simulink model "sf_multfuncout"  (Simulink 7.6)
settings: Solver=ode45  StartTime=0.0  StopTime=30  MaxStep=1  RelTol=1e-3
settings Model: Creator=The MathWorks Inc.  CovMetricSettings=dcmtr  ExtModeAutoUpdateStatusClock=off
settings OptimizationCC: BooleanDataType=off  InlineInvariantSignals=on  InitFltsAndDblsToZero=on  EfficientMapNaN2IntZero=off
settings DebuggingCC: SaveWithParameterizedLinksMsg=none  SignalResolutionControl=TryResolveAllWithWarning  SolverPrmCheckMsg=none  MultiTaskDSMMsg=warning  MultiTaskCondExecSysMsg=none  StrictBusMsg=None
settings HardwareCC: TargetUnknown=on
settings SFSimCC: SimParseCustomCode=off
settings RTWCC: IncludeERTFirstTime=on
settings GRTTargetCC: TargetFcnLib=ansi_tfl_tmw.mat

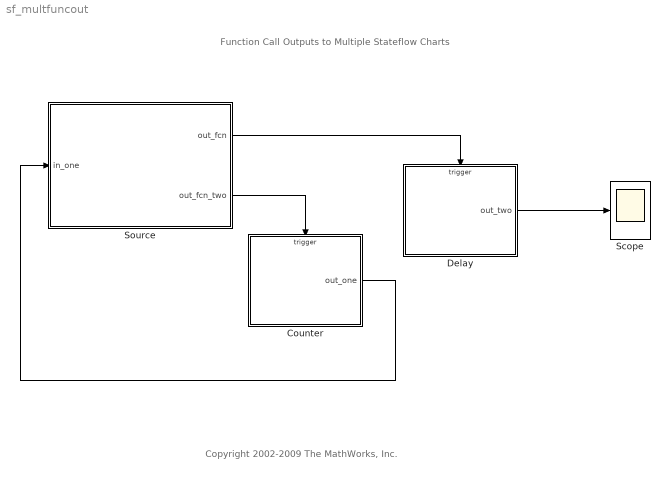
== system sf_multfuncout ==
  note: Function Call Outputs to Multiple Stateflow Charts
  note: Copyright 2002-2009 The MathWorks, Inc.
  Counter : Stateflow chart  TreatAsAtomicUnit=on
  Delay : Stateflow chart  TreatAsAtomicUnit=on
  Scope : Scope
      settings: TimeRange=30  YMin=0  YMax=7
  Source : Stateflow chart  TreatAsAtomicUnit=on
  wires:
  Source/2(out_fcn_two) -> Counter/Trigger
  Source/1(out_fcn) -> Delay/Trigger
  Delay/1(out_two) -> Scope/1
  Counter/1(out_one) -> Source/1(in_one)

== stateflow chart Source ==
  state A
  state B
  state C
  A -> B : /out_fcn_two;
  B -> A [order 2] : /out_fcn_two;
  (default) -> A
  B -> C [order 1] : [in_one>10]/out_fcn;
  C -> A
  data: in_one input double
  events: out_fcn output FUNCTION_CALL_EVENT; out_fcn_two output FUNCTION_CALL_EVENT

== stateflow chart Counter ==
  state A
    en:out_one=1;
    du:out_one++;
  (default) -> A
  data: out_one output double
  events: event input FUNCTION_CALL_EVENT

== stateflow chart Delay ==
  state A
    en:out_two=1;
    du:out_two++;
  (default) -> A
  data: out_two output double
  events: event input FUNCTION_CALL_EVENT
